simulink library "ebdc"  (Simulink 8.1)
settings: Solver=ode1  StartTime=0.0  StopTime=Inf  FixedStep=0.001  RelTol=1e-3
PostLoadFcn:
  | , if any(exist('dsrtsu_mdlpostloadfcn', 'file') == [2, 3, 6]), try dsrtsu_mdlpostloadfcn('Execute', bdroot); catch fprintf('Error in PostLoadFcn (dsrtsu_mdlpostloadfcn) for model "%s":\n %s\n', bdroot, lasterr); end, end,
settings Model: DSRTSU_INTERNAL_RTI_VER=450  DSRTSU_INTERNAL_RTI_TYPE=rti1401  Creator=tescamilla  LastModifiedBy=tescamilla

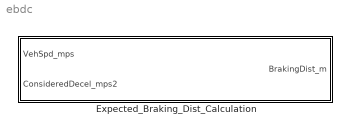
== system ebdc ==
  Expected_Braking_Dist_Calculation : Subsystem

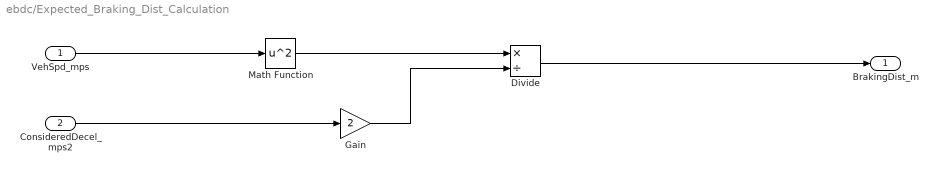
== system ebdc/Expected_Braking_Dist_Calculation ==
  VehSpd_mps : Inport
  ConsideredDecel_mps2 : Inport  Port=2
  Divide : Product  Inputs=*/
  Gain : Gain  Gain=2
  Math Function : Math  Operator=square  SaturateOnIntegerOverflow=on
  BrakingDist_m : Outport
  wires:
  ConsideredDecel_mps2/1 -> Gain/1
  Gain/1 -> Divide/2
  Divide/1 -> BrakingDist_m/1
  Math Function/1 -> Divide/1
  VehSpd_mps/1 -> Math Function/1
